simulink model "untitled1"  (R2015a)
settings: Solver=ode45  StartTime=0.0  StopTime=10.0  RelTol=1e-3
libraries: powerlib x13
settings Model: Creator=SELVA SAM  LastModifiedBy=SELVA SAM

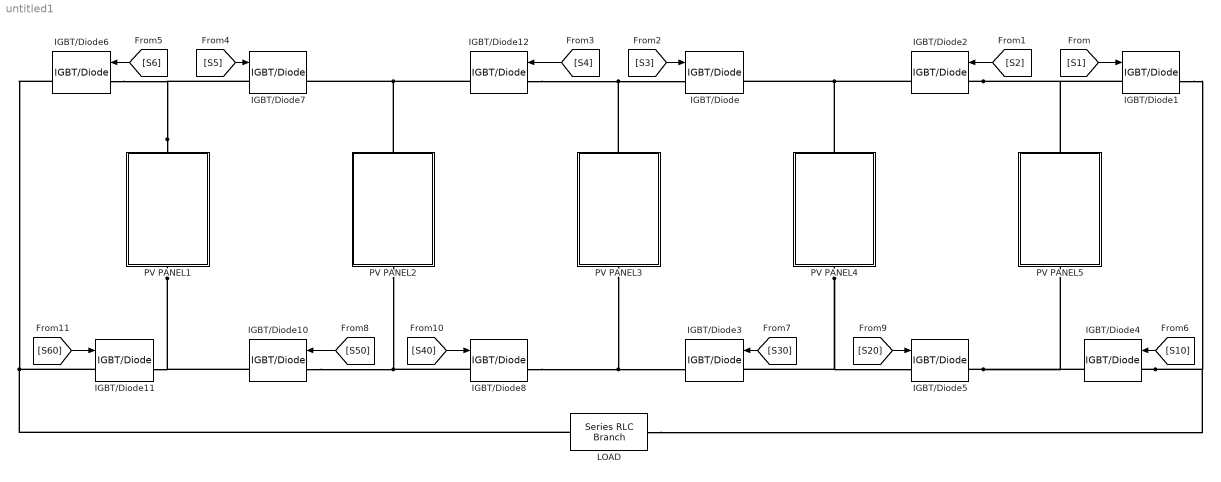
== system untitled1 ==
  IGBT/Diode{,1..8,10..12} (12 alike) : powerlib/Power Electronics/IGBT//Diode  Ron=1e-3  Rs=1e5  Cs=inf  Measurements=on
  "LOAD " : powerlib/Elements/Series RLC Branch  LConnTagsString=__new0  RConnTagsString=__new0  BranchType=R  Resistance=1  Inductance=1e-3  SetiL0=off  InitialCurrent=0  Capacitance=1e-6  Setx0=off  InitialVoltage=0  Measurements=None
  PV PANEL1 : Subsystem
      mask Display: image('C:\Users\SELVA SAM\Downloads\2.jpg')
  PV PANEL2 : Subsystem
      mask Display: image('C:\Users\SELVA SAM\Downloads\2.jpg')
  PV PANEL3 : Subsystem
      mask Display: image('C:\Users\SELVA SAM\Downloads\2.jpg')
  PV PANEL4 : Subsystem
      mask Display: image('C:\Users\SELVA SAM\Downloads\2.jpg')
  PV PANEL5 : Subsystem
      mask Display: image('C:\Users\SELVA SAM\Downloads\2.jpg')
  wires:
  [S1] -> IGBT/Diode1/1
  [S2] -> IGBT/Diode2/1
  [S4] -> IGBT/Diode12/1
  [S3] -> IGBT/Diode/1
  [S6] -> IGBT/Diode6/1
  [S5] -> IGBT/Diode7/1
  [S10] -> IGBT/Diode4/1
  [S30] -> IGBT/Diode3/1
  [S50] -> IGBT/Diode10/1
  [S20] -> IGBT/Diode5/1
  [S40] -> IGBT/Diode8/1
  [S60] -> IGBT/Diode11/1
  connections:
  PV PANEL4/LConn1 -- IGBT/Diode2/RConn1 -- IGBT/Diode/RConn1
  IGBT/Diode2/LConn1 -- IGBT/Diode1/LConn1 -- PV PANEL5/LConn1
  PV PANEL4/RConn1 -- IGBT/Diode5/LConn1 -- IGBT/Diode3/LConn1
  IGBT/Diode5/RConn1 -- IGBT/Diode4/RConn1 -- PV PANEL5/RConn1
  IGBT/Diode4/LConn1 -- "LOAD "/RConn1 -- IGBT/Diode1/RConn1
  PV PANEL1/LConn1 -- IGBT/Diode6/LConn1 -- IGBT/Diode7/LConn1
  PV PANEL2/LConn1 -- IGBT/Diode12/RConn1 -- IGBT/Diode7/RConn1
  PV PANEL1/RConn1 -- IGBT/Diode11/RConn1 -- IGBT/Diode10/RConn1
  IGBT/Diode10/LConn1 -- IGBT/Diode8/LConn1 -- PV PANEL2/RConn1
  IGBT/Diode12/LConn1 -- IGBT/Diode/LConn1 -- PV PANEL3/LConn1
  IGBT/Diode8/RConn1 -- IGBT/Diode3/RConn1 -- PV PANEL3/RConn1
  IGBT/Diode6/RConn1 -- "LOAD "/LConn1 -- IGBT/Diode11/LConn1

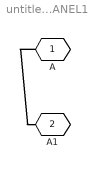
== system untitled1/PV PANEL1 ==
  A : PMIOPort  Port=1  Side=Left
  A1 : PMIOPort  Port=2  Side=Right
  connections:
  A/RConn1 -- A1/RConn1

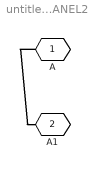
== system untitled1/PV PANEL2 ==
  A : PMIOPort  Port=1  Side=Left
  A1 : PMIOPort  Port=2  Side=Right
  connections:
  A/RConn1 -- A1/RConn1

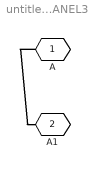
== system untitled1/PV PANEL3 ==
  A : PMIOPort  Port=1  Side=Left
  A1 : PMIOPort  Port=2  Side=Right
  connections:
  A/RConn1 -- A1/RConn1

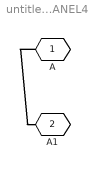
== system untitled1/PV PANEL4 ==
  A : PMIOPort  Port=1  Side=Left
  A1 : PMIOPort  Port=2  Side=Right
  connections:
  A/RConn1 -- A1/RConn1

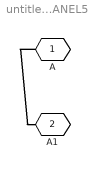
== system untitled1/PV PANEL5 ==
  A : PMIOPort  Port=1  Side=Left
  A1 : PMIOPort  Port=2  Side=Right
  connections:
  A/RConn1 -- A1/RConn1
